simulink model "flexible_shafts"  (R2025a)
settings: Solver=VariableStepAuto  StartTime=0.0  StopTime=simlength  RelTol=1e-3
values from neighbouring files (symbols this model uses):
  K = lqr(A,B,Q,R)    [init_msm.m]
  simlength = 30    [init_msm.m]
  Tc = Ts    (= 0.001)    [init_msm.m]
libraries: nesl_utility x6, fl_lib x3, flexshaft_2masses_lib x1
settings Model: Creator=dbagn  LastModifiedBy=dbagn
settings DataIOCC: SaveOutput=off  SignalLogging=off  DSMLogging=off  SaveTime=off  ReturnWorkspaceOutputs=off

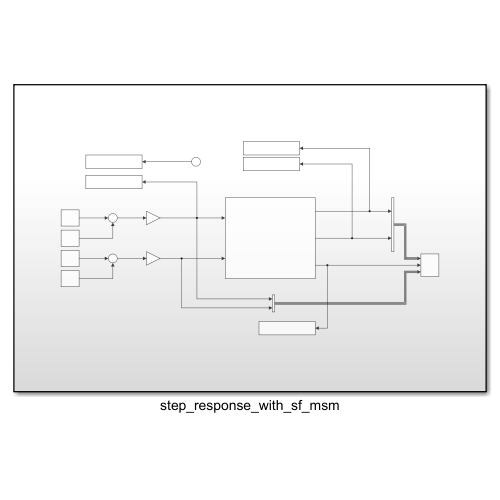
[thumbnail: Simulink's stored preview of the top-level diagram]
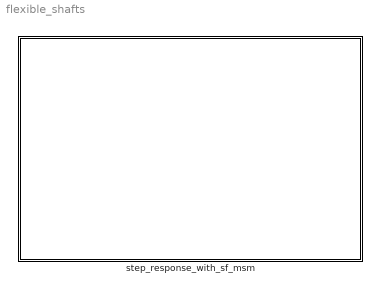
== system flexible_shafts ==
  step_response_with_sf_msm : Subsystem

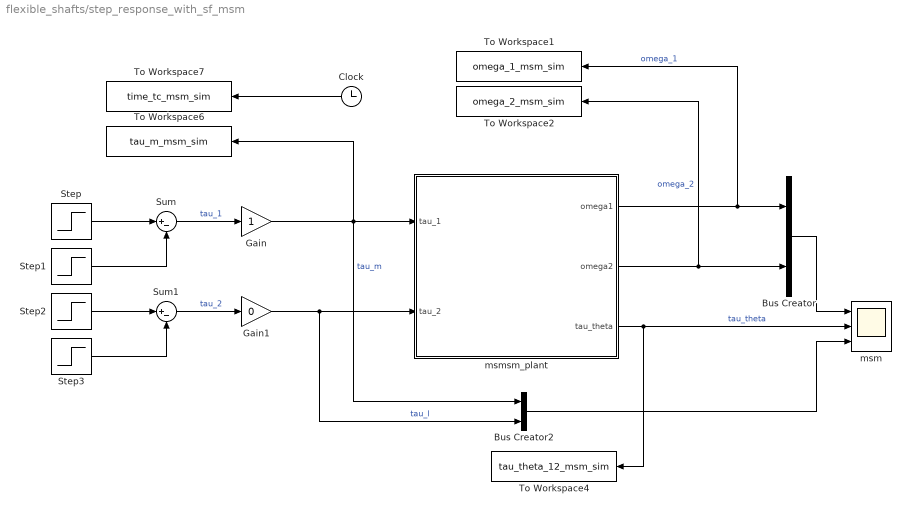
== system flexible_shafts/step_response_with_sf_msm ==
  Bus Creator : BusCreator  Inputs=2
  Bus Creator2 : BusCreator  Inputs=2
  Clock : Clock
  Gain : Gain
  Gain1 : Gain  Gain=0
  Step : Step  Time=0.2  SampleTime=0
  Step1 : Step  Time=0.25  SampleTime=0
  Step2 : Step  Time=0.2+simlength/2  SampleTime=0
  Step3 : Step  Time=0.25+simlength/2  SampleTime=0
  Sum : Sum  Inputs=|+-
  Sum1 : Sum  Inputs=|+-
  To Workspace1 : ToWorkspace  VariableName=omega_1_msm_sim  SampleTime=Tc
      settings: MaxDataPoints=Nc
  To Workspace2 : ToWorkspace  VariableName=omega_2_msm_sim  SampleTime=Tc
      settings: MaxDataPoints=Nc
  To Workspace4 : ToWorkspace  VariableName=tau_theta_12_msm_sim  SampleTime=Tc
      settings: MaxDataPoints=Nc
  To Workspace6 : ToWorkspace  VariableName=tau_m_msm_sim  SampleTime=Tc
      settings: MaxDataPoints=Nc
  To Workspace7 : ToWorkspace  VariableName=time_tc_msm_sim  SampleTime=Tc
      settings: MaxDataPoints=Nc
  msm : Scope  NumInputPorts=3
      settings: SampleTime=Tc  ActiveDisplayYMinimum=-0.435306587887276  ActiveDisplayYMaximum=0.34041406759201609
  msmsm_plant : Subsystem
  wires:
  msmsm_plant/1(omega1) -> To Workspace1/1, Bus Creator/1  "omega_1"
  Clock/1 -> To Workspace7/1
  msmsm_plant/2(omega2) -> To Workspace2/1, Bus Creator/2  "omega_2"
  Gain/1 -> To Workspace6/1, msmsm_plant/1(tau_1), Bus Creator2/1  "tau_m"
  Bus Creator2/1 -> msm/3
  msmsm_plant/3(tau_theta) -> msm/2, To Workspace4/1  "tau_theta"
  Bus Creator/1 -> msm/1
  Step2/1 -> Sum1/1
  Sum1/1 -> Gain1/1  "tau_2"
  Step3/1 -> Sum1/2
  Sum/1 -> Gain/1  "tau_1"
  Step/1 -> Sum/1
  Step1/1 -> Sum/2
  Gain1/1 -> msmsm_plant/2(tau_2), Bus Creator2/2  "tau_l"

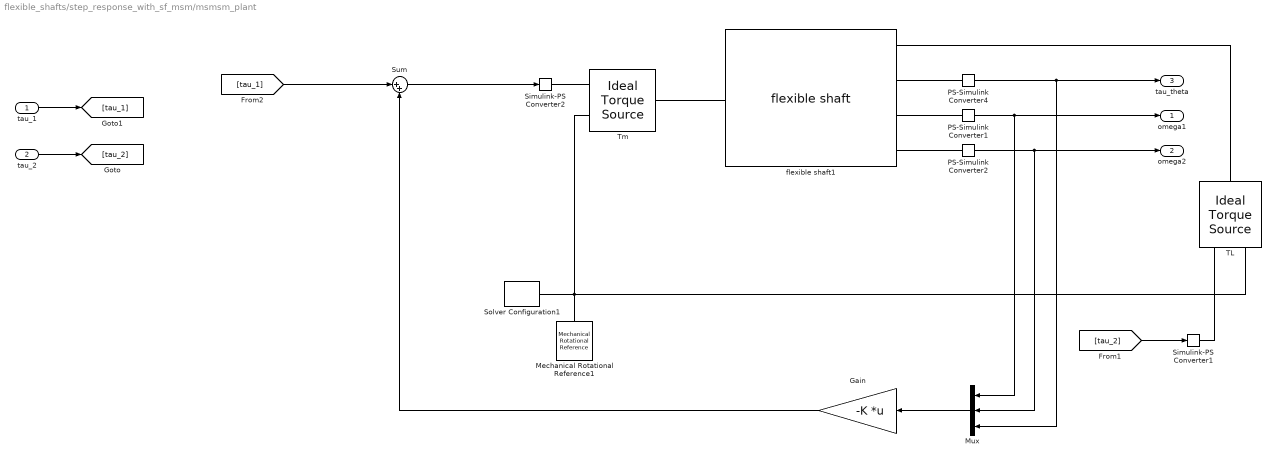
== system flexible_shafts/step_response_with_sf_msm/msmsm_plant ==
  tau_1 : Inport
  tau_2 : Inport  Port=2
  Gain : Gain  Gain=-K  Multiplication=Matrix(K*u)
  Mechanical Rotational Reference1 : fl_lib/Mechanical/Rotational Elements/Mechanical Rotational Reference
  Mux : Mux  Inputs=3
  PS-Simulink Converter1 : nesl_utility/PS-Simulink Converter  PhysicalDomain=network_engine_domain  SubClassName=ps_output  LeftPortType=input  RightPortType=output  PseudoPeriodic=off  Frequencies=[]  VectorFormat=1-D array  Unit=1  AffineConversion=off
  PS-Simulink Converter2 : nesl_utility/PS-Simulink Converter  PhysicalDomain=network_engine_domain  SubClassName=ps_output  LeftPortType=input  RightPortType=output  PseudoPeriodic=off  Frequencies=[]  VectorFormat=1-D array  Unit=1  AffineConversion=off
  PS-Simulink Converter4 : nesl_utility/PS-Simulink Converter  PhysicalDomain=network_engine_domain  SubClassName=ps_output  LeftPortType=input  RightPortType=output  PseudoPeriodic=off  Frequencies=[]  VectorFormat=1-D array  Unit=1  AffineConversion=off
  Simulink-PS Converter1 : nesl_utility/Simulink-PS Converter  PhysicalDomain=network_engine_domain  SubClassName=ps_input  LeftPortType=input  RightPortType=output  PseudoPeriodic=off  Frequencies=[]  NoiseDistribution=none  NoiseParameters=[]  Unit=1  AffineConversion=off  FilteringAndDerivatives=provide  SimscapeFilterOrder=1  InputFilterTimeConstant=0.001  UdotUserProvided=0
  Simulink-PS Converter2 : nesl_utility/Simulink-PS Converter  PhysicalDomain=network_engine_domain  SubClassName=ps_input  LeftPortType=input  RightPortType=output  PseudoPeriodic=off  Frequencies=[]  NoiseDistribution=none  NoiseParameters=[]  Unit=1  AffineConversion=off  FilteringAndDerivatives=provide  SimscapeFilterOrder=1  InputFilterTimeConstant=0.001  UdotUserProvided=0
  Solver Configuration1 : nesl_utility/Solver Configuration  PhysicalDomain=network_engine_domain  SubClassName=solver  LeftPortType=input  RightPortType=generic  Tones=[]  Harmonics=[]  SimulateNoise=off  Profile=off  UseLocalSampling=off  EnableSwitchedLinearOptims=on  FrequencyDomain=off  UseCCode=off  RelTol=0.001  AbsTol=1e-06  MinStep=1e-09  ToWorkspace=off  RevertToSquareIcSolve=off  NumHomotopyIterations=100  PhasorMode=off  PhasorModeNumHarmonics=1  ConsistencySolver=NEWTON_FTOL  IndexReductionMethod=DerivativeReplacement  DoDC=off  ResidualTolerance=1e-09  ConsistencyTolSource=GLOBAL  ConsistencyAbsTol=0.001  ConsistencyRelTol=0.001  ConsistencyTolFactor=0.001  UseLocalSolver=off  LocalSolverChoice=NE_BACKWARD_EULER_ADVANCER  ResolveIndetEquations=on  FunctionEvalNumThread=1  LocalSolverSampleTime=0.001  DoFixedCost=off  MaxNonlinIter=3  MaxModeIter=2  ComputeImpulses=off  ImpulseIterations=2  LinearAlgebra=auto  LinearAlgebraNumThread=0  EquationFormulation=NE_TIME_EF  DelaysMemoryBudget=1024  AutomaticFiltering=on  FilteringTimeConstant=0.001  PartitionStorageMethod=AS_NEEDED  PartitionMemoryBudget=1024  PartitionMethod=ROBUST  MultibodyUseLocalSolver=off  MultibodyLocalSolverChoice=ODE1  MultibodyLocalSolverSampleTime=0.001
  Sum : Sum  Inputs=|++
  TL : fl_lib/Mechanical/Mechanical Sources/Ideal Torque Source
  "Tm " : fl_lib/Mechanical/Mechanical Sources/Ideal Torque Source
  flexible shaft1 : flexshaft_2masses_lib/flexible shaft  b1=b1 N*m*s/rad  J1=J1 kg*m^2  b2=b2 N*m*s/rad  J2=J2 kg*m^2  b_theta=b_theta N*m*s/rad  k_theta=k_theta N*m/rad  w_1_specify=off  w_1_priority=None  w_1=0 rad/s  w_1_nominal_specify=off  w_1_nominal_value=1  w_1_nominal_unit=rad/s  w_2_specify=off  w_2_priority=None  w_2=0 rad/s  w_2_nominal_specify=off  w_2_nominal_value=1  w_2_nominal_unit=rad/s  t_1_specify=off  t_1_priority=None  t_1=0 N*m  t_1_nominal_specify=off  t_1_nominal_value=1  t_1_nominal_unit=N*m  t_2_specify=off  t_2_priority=None  t_2=0 N*m  t_2_nominal_specify=off  t_2_nominal_value=1  t_2_nominal_unit=N*m  t_theta_specify=off  t_theta_priority=None  t_theta=0 N*m  t_theta_nominal_specify=off  t_theta_nominal_value=1  t_theta_nominal_unit=N*m
      settings: InternalSimscapePortConfiguration="{\"Bottom\":[],\"Left\":[{\"id\":\"S1\",\"label\":\"S1\",\"type\":\"foundation.mechanical.rotational.rotational\"}],\"Right\":[{\"id\":\"S2\",\"label\":\"S2\",\"type\":\"foundation.mechanical.rotational.rotational\"},{\"id\":\"tau_theta\",\"label\":\"tau_theta\",\"type\":\"output\"},{\"id\":\"w1\",\"label\":\"w1\",\"type\":\"output\"},{\"id\":\"w2\",\"label\":\"w2\",\"type\":\"output\"}],\"Top\":[]}"
  omega1 : Outport
  omega2 : Outport  Port=2
  tau_theta : Outport  Port=3
  wires:
  PS-Simulink Converter1/1 -> omega1/1, Mux/1
  PS-Simulink Converter2/1 -> omega2/1, Mux/2
  PS-Simulink Converter4/1 -> tau_theta/1, Mux/3
  tau_1/1 -> [tau_1]
  tau_2/1 -> [tau_2]
  [tau_2] -> Simulink-PS Converter1/1
  Mux/1 -> Gain/1
  Sum/1 -> Simulink-PS Converter2/1
  [tau_1] -> Sum/1
  Gain/1 -> Sum/2
  connections:
  PS-Simulink Converter4/LConn1 -- flexible shaft1/RConn2
  Simulink-PS Converter2/RConn1 -- "Tm "/RConn1
  flexible shaft1/LConn1 -- "Tm "/LConn1
  Simulink-PS Converter1/RConn1 -- TL/RConn1
  TL/LConn1 -- flexible shaft1/RConn1
  Solver Configuration1/RConn1 -- Mechanical Rotational Reference1/LConn1 -- "Tm "/RConn2 -- TL/RConn2
  PS-Simulink Converter1/LConn1 -- flexible shaft1/RConn3
  flexible shaft1/RConn4 -- PS-Simulink Converter2/LConn1
